simulink model "SYSTEM"  (R2026a)
settings: Solver=VariableStepAuto
model workspace (MAT data in the model file):
  CompAir_P = Simulink.ConnectionBus
  CompAir_S = Simulink.Bus
  CompAir_S.Alignment = -1
  CompAir_S.PreserveElementDimensions = 0
  CompAir_S.DataScope = 'Auto'
  Control_P = Simulink.ConnectionBus
  Control_S = Simulink.Bus
  Control_S.Alignment = -1
  Control_S.PreserveElementDimensions = 0
  Control_S.DataScope = 'Auto'
  CoolingFW_P = Simulink.ConnectionBus
  CoolingFW_S = Simulink.Bus
  CoolingFW_S.Alignment = -1
  CoolingFW_S.PreserveElementDimensions = 0
  CoolingFW_S.DataScope = 'Auto'
  FuelOil_P = Simulink.ConnectionBus
  FuelOil_S = Simulink.Bus
  FuelOil_S.Alignment = -1
  FuelOil_S.PreserveElementDimensions = 0
  FuelOil_S.DataScope = 'Auto'
  Heat_P = Simulink.ConnectionBus
  Heat_S = Simulink.Bus
  Heat_S.Alignment = -1
  Heat_S.PreserveElementDimensions = 0
  Heat_S.DataScope = 'Auto'
  LubeOil_P = Simulink.ConnectionBus
  LubeOil_S = Simulink.Bus
  LubeOil_S.Alignment = -1
  LubeOil_S.PreserveElementDimensions = 0
  LubeOil_S.DataScope = 'Auto'
  Physical = Simulink.ConnectionBus
  Power_P = Simulink.ConnectionBus
  Power_S = Simulink.Bus
  Power_S.Alignment = -1
  Power_S.PreserveElementDimensions = 0
  Power_S.DataScope = 'Auto'
  SaltWater_P = Simulink.ConnectionBus
  SaltWater_S = Simulink.Bus
  SaltWater_S.Alignment = -1
  SaltWater_S.PreserveElementDimensions = 0
  SaltWater_S.DataScope = 'Auto'
  WasteGas_P = Simulink.ConnectionBus
  WasteGas_S = Simulink.Bus
  WasteGas_S.Alignment = -1
  WasteGas_S.PreserveElementDimensions = 0
  WasteGas_S.DataScope = 'Auto'
  WasteOil_P = Simulink.ConnectionBus
  WasteOil_S = Simulink.Bus
  WasteOil_S.Alignment = -1
  WasteOil_S.PreserveElementDimensions = 0
  WasteOil_S.DataScope = 'Auto'
  WasteSolid_P = Simulink.ConnectionBus
  WasteSolid_S = Simulink.Bus
  WasteSolid_S.Alignment = -1
  WasteSolid_S.PreserveElementDimensions = 0
  WasteSolid_S.DataScope = 'Auto'
  WasteWater_P = Simulink.ConnectionBus
  WasteWater_S = Simulink.Bus
  WasteWater_S.Alignment = -1
  WasteWater_S.PreserveElementDimensions = 0
  WasteWater_S.DataScope = 'Auto'
undefined symbols (not defined in the file): FUEL
(part 1 of 5)
settings Model: VariantConfigurationObject=ConfigA  Creator=GShelton28  LastModifiedBy=sboyd

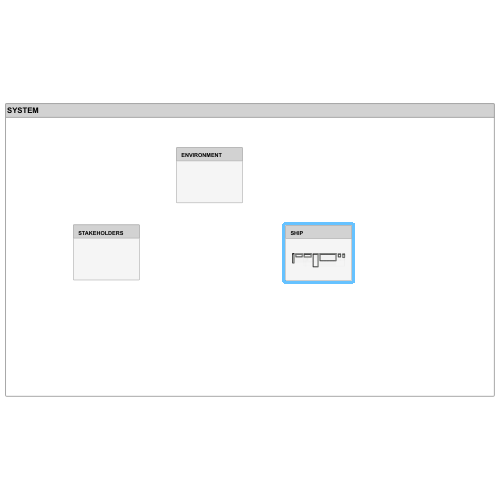
[thumbnail: Simulink's stored preview of the top-level diagram]
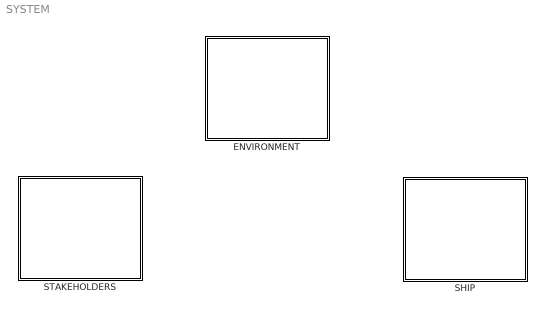
== system SYSTEM ==
  ENVIRONMENT : Subsystem
      settings: PortSchema="{\"entries\":[{\"content\":{\"headerSize\":26,\"margin\":15,\"minimumSpacing\":25,\"sides\":[{\"content\":{},\"type\":\"ConnectorPlacement.EquallySpacedRectSide\",\"uuid\":\"c62bca68-e99b-4d4a-8c3b-c9a3c6520291\"},{\"content\":{\"side\":\"RIGHT\"},\"type\":\"ConnectorPlacement.EquallySpacedRectSide\",\"uuid\":\"9f78cd75-5645-4950-8d66-9f0d33627f1f\"},{\"content\":{\"side\":\"TOP\"},\"type\":\"ConnectorPlacement.EquallySpacedRectSide\",\"uuid\":\"f95077c9-4a6b-4bf1-8b13-59697d659817\"}]},\"type\":\"ConnectorPlacement.EquallySpacedConnector\",\"uuid\":\"da1ef182-4ed3-4fb4-823f-e8eb0a5ecd15\"}],\"packageUris\":[\"http://schema.mathworks.com/mf0/Connector/R2020b\"],\"version\":\"1.0\"}"
  SHIP : Subsystem
      settings: PortSchema="{\"entries\":[{\"content\":{\"headerSize\":26,\"margin\":15,\"minimumSpacing\":25,\"sides\":[{\"content\":{},\"type\":\"ConnectorPlacement.EquallySpacedRectSide\",\"uuid\":\"c62bca68-e99b-4d4a-8c3b-c9a3c6520291\"},{\"content\":{\"side\":\"RIGHT\"},\"type\":\"ConnectorPlacement.EquallySpacedRectSide\",\"uuid\":\"9f78cd75-5645-4950-8d66-9f0d33627f1f\"},{\"content\":{\"side\":\"TOP\"},\"type\":\"ConnectorPlacement.EquallySpacedRectSide\",\"uuid\":\"f95077c9-4a6b-4bf1-8b13-59697d659817\"}]},\"type\":\"ConnectorPlacement.EquallySpacedConnector\",\"uuid\":\"da1ef182-4ed3-4fb4-823f-e8eb0a5ecd15\"}],\"packageUris\":[\"http://schema.mathworks.com/mf0/Connector/R2020b\"],\"version\":\"1.0\"}"
  STAKEHOLDERS : Subsystem
      settings: PortSchema="{\"entries\":[{\"content\":{\"headerSize\":26,\"margin\":15,\"minimumSpacing\":25,\"sides\":[{\"content\":{},\"type\":\"ConnectorPlacement.EquallySpacedRectSide\",\"uuid\":\"c62bca68-e99b-4d4a-8c3b-c9a3c6520291\"},{\"content\":{\"side\":\"RIGHT\"},\"type\":\"ConnectorPlacement.EquallySpacedRectSide\",\"uuid\":\"9f78cd75-5645-4950-8d66-9f0d33627f1f\"},{\"content\":{\"side\":\"TOP\"},\"type\":\"ConnectorPlacement.EquallySpacedRectSide\",\"uuid\":\"f95077c9-4a6b-4bf1-8b13-59697d659817\"}]},\"type\":\"ConnectorPlacement.EquallySpacedConnector\",\"uuid\":\"da1ef182-4ed3-4fb4-823f-e8eb0a5ecd15\"}],\"packageUris\":[\"http://schema.mathworks.com/mf0/Connector/R2020b\"],\"version\":\"1.0\"}"

== system SYSTEM/ENVIRONMENT ==

== system SYSTEM/SHIP ==
  100 (HULL) : Subsystem
      settings: PortSchema="{\"entries\":[{\"content\":{\"headerSize\":26,\"margin\":15,\"minimumSpacing\":25,\"sides\":[{\"content\":{},\"type\":\"ConnectorPlacement.EquallySpacedRectSide\",\"uuid\":\"c62bca68-e99b-4d4a-8c3b-c9a3c6520291\"},{\"content\":{\"connectorIds\":[\"RConn1\",\"RConn2\",\"RConn3\",\"RConn4\",\"RConn5\",\"RConn6\",\"RConn7\",\"RConn8\",\"RConn9\",\"RConn10\",\"RConn11\",\"RConn12\",\"RConn13\",\"RConn14\",\"RConn15\",\"RConn16\",\"RConn17\",\"RConn18\",\"RConn19\",\"RConn20\",\"RConn21\",\"RConn22\",\"RConn23\",\"RConn24\",\"RConn25\",\"RConn26\",\"RConn27\",\"RConn28\",\"RConn29\",\"RConn30\",\"RConn31\",\"RConn32\"],\"side\":\"RIGHT\"},\"type\":\"ConnectorPlacement.EquallySpacedRectSide\",\"uuid\":\"9f78cd75-5645-4950-8d66-9f0d33627f1f\"},{\"content\":{\"side\":\"TOP\"},\"type\":\"ConnectorPlacement.EquallySpacedRectSide\",\"uuid\":\"f95077c9-4a6b-4bf1-8b13-59697d659817\"}]},\"type\":\"ConnectorPlacement.EquallySpacedConnector\",\"uuid\":\"da1ef182-4ed3-4fb4-823f-e8eb0a5ecd15\"}],\"packageUris\":[\"http://schema.mathworks.com/mf0/Connector/R2020b\"],\"version\":\"1.0\"}"
  200 (PROPULSION) : Subsystem
      settings: PortSchema="{\"entries\":[{\"content\":{\"headerSize\":26,\"margin\":15,\"minimumSpacing\":25,\"sides\":[{\"content\":{\"connectorIds\":[\"LConn3\",\"LConn4\",\"LConn5\",\"LConn6\"]},\"type\":\"ConnectorPlacement.EquallySpacedRectSide\",\"uuid\":\"c62bca68-e99b-4d4a-8c3b-c9a3c6520291\"},{\"content\":{\"connectorIds\":[\"In11\",\"In12\",\"In13\",\"Out12\",\"Out13\",\"Out14\",\"Out15\"],\"side\":\"RIGHT\"},\"type\":\"ConnectorPlacement.EquallySpacedRectSide\",\"uuid\":\"9f78cd75-5645-4950-8d66-9f0d33627f1f\"},{\"content\":{\"connectorIds\":[\"Out1\",\"Out2\",\"Out3\",\"LConn1\",\"Out4\",\"Out5\",\"Out6\",\"Out7\",\"Out8\",\"Out9\",\"Out10\",\"Out11\",\"In1\",\"In2\",\"In3\",\"In4\",\"In5\",\"In6\",\"In7\",\"LConn2\",\"In8\",\"In9\",\"In10\"],\"side\":\"TOP\"},\"type\":\"ConnectorPlacement.EquallySpacedRectSide\",\"uuid\":\"f95077c9-4a6b-4bf1-8b13-59697d659817\"},{\"content\":{\"connectorIds\":[\"Out16\"],\"side\":\"BOTTOM\"},\"type\":\"ConnectorPlacement.EquallySpacedRectSide\",\"uuid\":\"7ad02fd3-1470-4b5e-9c8f-1c514025d559\"}]},\"type\":\"ConnectorPlacement.EquallySpacedConnector\",\"uuid\":\"da1ef182-4ed3-4fb4-823f-e8eb0a5ecd15\"}],\"packageUris\":[\"http://schema.mathworks.com/mf0/Connector/R2020b\"],\"version\":\"1.0\"}"
  300 (ELECTRICAL) : Subsystem
      settings: PortSchema="{\"entries\":[{\"content\":{\"headerSize\":26,\"margin\":15,\"minimumSpacing\":25,\"sides\":[{\"content\":{\"connectorIds\":[\"LConn3\",\"LConn4\",\"LConn5\",\"LConn6\"]},\"type\":\"ConnectorPlacement.EquallySpacedRectSide\",\"uuid\":\"c62bca68-e99b-4d4a-8c3b-c9a3c6520291\"},{\"content\":{\"connectorIds\":[\"In5\",\"In6\",\"In7\",\"In8\",\"Out6\",\"Out7\",\"Out8\",\"Out9\"],\"side\":\"RIGHT\"},\"type\":\"ConnectorPlacement.EquallySpacedRectSide\",\"uuid\":\"9f78cd75-5645-4950-8d66-9f0d33627f1f\"},{\"content\":{\"connectorIds\":[\"Out1\",\"Out2\",\"Out3\",\"LConn1\",\"Out4\",\"Out5\",\"In1\",\"In2\",\"In3\",\"LConn2\",\"In4\"],\"side\":\"TOP\"},\"type\":\"ConnectorPlacement.EquallySpacedRectSide\",\"uuid\":\"f95077c9-4a6b-4bf1-8b13-59697d659817\"},{\"content\":{\"connectorIds\":[\"In9\",\"Out10\",\"Out11\",\"Out12\",\"Out13\",\"Out14\",\"Out15\",\"Out16\",\"Out17\",\"Out18\",\"Out19\",\"Out20\",\"Out21\",\"Out22\",\"Out23\",\"Out24\",\"Out25\",\"Out26\",\"Out27\",\"Out28\",\"Out29\",\"Out30\",\"Out31\",\"Out32\"],\"side\":\"BOTTOM\"},\"type\":\"ConnectorPlacement.EquallySpacedRectSide\",\"uuid\":\"f64e9209-9b7e-40f6-99bd-cc5d8e42f30b\"}]},\"type\":\"ConnectorPlacement.EquallySpacedConnector\",\"uuid\":\"da1ef182-4ed3-4fb4-823f-e8eb0a5ecd15\"}],\"packageUris\":[\"http://schema.mathworks.com/mf0/Connector/R2020b\"],\"version\":\"1.0\"}"
  400 (COMMAND CONTROL) : Subsystem
      settings: PortSchema="{\"entries\":[{\"content\":{\"headerSize\":26,\"margin\":15,\"minimumSpacing\":25,\"sides\":[{\"content\":{\"connectorIds\":[\"LConn1\",\"LConn2\",\"LConn3\",\"LConn4\",\"LConn5\",\"LConn6\"]},\"type\":\"ConnectorPlacement.EquallySpacedRectSide\",\"uuid\":\"c62bca68-e99b-4d4a-8c3b-c9a3c6520291\"},{\"content\":{\"connectorIds\":[\"In10\",\"In11\",\"In12\",\"In13\",\"In6\",\"In7\",\"In8\",\"In9\",\"In14\",\"In15\",\"In16\",\"In17\",\"In18\",\"In19\",\"In20\",\"In21\",\"In22\",\"In23\",\"In24\",\"In25\",\"In26\",\"In27\",\"In28\",\"Out6\",\"Out7\",\"Out8\",\"Out9\",\"Out10\",\"Out11\",\"Out12\",\"Out13\",\"Out14\",\"Out15\",\"Out16\",\"Out17\",\"Out18\",\"Out19\",\"Out20\",\"Out21\",\"Out22\",\"Out23\",\"Out24\",\"Out25\",\"Out26\",\"Out27\"],\"side\":\"RIGHT\"},\"type\":\"ConnectorPlacement.EquallySpacedRectSide\",\"uuid\":\"9f78cd75-5645-4950-8d66-9f0d33627f1f\"},{\"content\":{\"connectorIds\":[\"Out1\",\"Out3\",\"Out2\",\"Out4\",\"Out5\",\"In1\",\"In3\",\"In2\",\"In4\",\"In5\"],\"side\":\"TOP\"},\"type\":\"ConnectorPlacement.EquallySpacedRectSide\",\"uuid\":\"f95077c9-4a6b-4bf1-8b13-59697d659817\"},{\"content\":{\"connectorIds\":[\"In29\",\"In30\",\"In31\",\"In32\",\"In33\",\"In34\"],\"side\":\"BOTTOM\"},\"type\":\"ConnectorPlacement.EquallySpacedRectSide\",\"uuid\":\"b87ed66e-141b-41a3-a484-184f926198b1\"}]},\"type\":\"ConnectorPlacement.EquallySpacedConnector\",\"uuid\":\"da1ef182-4ed3-4fb4-823f-e8eb0a5ecd15\"}],\"packageUris\":[\"http://schema.mathworks.com/mf0/Connector/R2020b\"],\"version\":\"1.0\"}"
  500 (AUXILLIARY SYSTEMS) : Subsystem
      settings: PortSchema="{\"entries\":[{\"content\":{\"headerSize\":26,\"margin\":15,\"minimumSpacing\":25,\"sides\":[{\"content\":{\"connectorIds\":[\"LConn5\",\"LConn6\",\"LConn7\",\"LConn8\",\"LConn9\",\"LConn10\",\"LConn11\",\"LConn12\",\"LConn13\",\"LConn14\"]},\"type\":\"ConnectorPlacement.EquallySpacedRectSide\",\"uuid\":\"c62bca68-e99b-4d4a-8c3b-c9a3c6520291\"},{\"content\":{\"connectorIds\":[\"In31\",\"In32\",\"In33\",\"In34\",\"In35\",\"In36\",\"In37\",\"In38\",\"In39\",\"In40\",\"In41\",\"In42\",\"Out25\",\"Out26\",\"Out27\",\"Out28\",\"Out29\",\"Out30\",\"Out31\",\"Out32\",\"Out33\",\"Out34\",\"Out35\",\"Out36\"],\"side\":\"RIGHT\"},\"type\":\"ConnectorPlacement.EquallySpacedRectSide\",\"uuid\":\"9f78cd75-5645-4950-8d66-9f0d33627f1f\"},{\"content\":{\"connectorIds\":[\"Out1\",\"Out2\",\"Out3\",\"Out4\",\"Out5\",\"Out6\",\"Out7\",\"Out8\",\"Out9\",\"Out10\",\"Out11\",\"Out12\",\"Out13\",\"Out14\",\"Out15\",\"Out16\",\"Out17\",\"Out18\",\"LConn1\",\"Out19\",\"LConn2\",\"Out20\",\"Out21\",\"Out22\",\"Out23\",\"Out24\",\"In1\",\"In25\",\"In3\",\"LConn3\",\"In4\",\"In5\",\"In2\",\"In28\",\"In8\",\"In29\",\"In10\",\"In30\",\"In6\",\"In13\",\"In14\",\"LConn4\",\"In15\",\"In16\",\"In17\",\"In7\",\"In9\",\"In20\",\"In11\",\"In12\",\"In23\",\"In24\",\"In22\",\"In26\",\"In27\",\"In19\",\"In21\",\"In18\"],\"side\":\"TOP\"},\"type\":\"ConnectorPlacement.EquallySpacedRectSide\",\"uuid\":\"f95077c9-4a6b-4bf1-8b13-59697d659817\"},{\"content\":{\"connectorIds\":[\"In43\",\"In44\",\"In45\",\"In46\",\"In47\",\"In48\",\"In49\",\"In50\",\"In51\",\"In52\"],\"side\":\"BOTTOM\"},\"type\":\"ConnectorPlacement.EquallySpacedRectSide\",\"uuid\":\"1e4b81d9-ad89-4d5a-adb7-9dee60647f33\"}]},\"type\":\"ConnectorPlacement.EquallySpacedConnector\",\"uuid\":\"da1ef182-4ed3-4fb4-823f-e8eb0a5ecd15\"}],\"packageUris\":[\"http://schema.mathworks.com/mf0/Connector/R2020b\"],\"version\":\"1.0\"}"
  600 (OUTFITTING) : Subsystem
      settings: PortSchema="{\"entries\":[{\"content\":{\"headerSize\":26,\"margin\":15,\"minimumSpacing\":25,\"sides\":[{\"content\":{\"connectorIds\":[\"LConn1\",\"LConn2\",\"LConn3\"]},\"type\":\"ConnectorPlacement.EquallySpacedRectSide\",\"uuid\":\"c62bca68-e99b-4d4a-8c3b-c9a3c6520291\"},{\"content\":{\"connectorIds\":[\"In3\",\"In4\",\"Out7\",\"Out8\"],\"side\":\"RIGHT\"},\"type\":\"ConnectorPlacement.EquallySpacedRectSide\",\"uuid\":\"9f78cd75-5645-4950-8d66-9f0d33627f1f\"},{\"content\":{\"connectorIds\":[\"Out1\",\"Out2\",\"Out3\",\"Out4\",\"Out5\",\"Out6\",\"In1\",\"In2\"],\"side\":\"TOP\"},\"type\":\"ConnectorPlacement.EquallySpacedRectSide\",\"uuid\":\"f95077c9-4a6b-4bf1-8b13-59697d659817\"},{\"content\":{\"connectorIds\":[\"In5\",\"In6\"],\"side\":\"BOTTOM\"},\"type\":\"ConnectorPlacement.EquallySpacedRectSide\",\"uuid\":\"1c2b3604-2b1a-4429-bb6b-614e1a01ce36\"}]},\"type\":\"ConnectorPlacement.EquallySpacedConnector\",\"uuid\":\"da1ef182-4ed3-4fb4-823f-e8eb0a5ecd15\"}],\"packageUris\":[\"http://schema.mathworks.com/mf0/Connector/R2020b\"],\"version\":\"1.0\"}"
  700 (WEAPONS) : Subsystem
      settings: PortSchema="{\"entries\":[{\"content\":{\"headerSize\":26,\"margin\":15,\"minimumSpacing\":25,\"sides\":[{\"content\":{\"connectorIds\":[\"LConn1\",\"LConn2\",\"LConn3\",\"LConn4\",\"LConn5\"]},\"type\":\"ConnectorPlacement.EquallySpacedRectSide\",\"uuid\":\"c62bca68-e99b-4d4a-8c3b-c9a3c6520291\"},{\"content\":{\"connectorIds\":[\"In4\",\"In5\",\"In6\",\"In7\",\"In8\",\"Out4\",\"Out5\",\"Out6\",\"Out7\",\"Out8\"],\"side\":\"RIGHT\"},\"type\":\"ConnectorPlacement.EquallySpacedRectSide\",\"uuid\":\"9f78cd75-5645-4950-8d66-9f0d33627f1f\"},{\"content\":{\"connectorIds\":[\"Out1\",\"Out2\",\"Out3\",\"In1\",\"In2\",\"In3\"],\"side\":\"TOP\"},\"type\":\"ConnectorPlacement.EquallySpacedRectSide\",\"uuid\":\"f95077c9-4a6b-4bf1-8b13-59697d659817\"},{\"content\":{\"connectorIds\":[\"In9\",\"In10\",\"In11\",\"In12\",\"In13\"],\"side\":\"BOTTOM\"},\"type\":\"ConnectorPlacement.EquallySpacedRectSide\",\"uuid\":\"b18ac05c-61d0-41e7-b1c6-0cdd3a4fef39\"}]},\"type\":\"ConnectorPlacement.EquallySpacedConnector\",\"uuid\":\"da1ef182-4ed3-4fb4-823f-e8eb0a5ecd15\"}],\"packageUris\":[\"http://schema.mathworks.com/mf0/Connector/R2020b\"],\"version\":\"1.0\"}"
  wires:
  200 (PROPULSION)/16(23X-31XP) -> 300 (ELECTRICAL)/9(23X-31XP)
  300 (ELECTRICAL)/10(31X-40XP) -> 400 (COMMAND CONTROL)/29(31X-40XP)
  300 (ELECTRICAL)/11(31X-41XP) -> 400 (COMMAND CONTROL)/30(31X-41XP)
  300 (ELECTRICAL)/12(31X-42XP) -> 400 (COMMAND CONTROL)/31(31X-42XP)
  300 (ELECTRICAL)/13(31X-43XP) -> 400 (COMMAND CONTROL)/32(31X-43XP)
  300 (ELECTRICAL)/14(31X-44XP) -> 400 (COMMAND CONTROL)/33(31X-44XP)
  300 (ELECTRICAL)/15(31X-45XP) -> 400 (COMMAND CONTROL)/34(31X-45XP)
  300 (ELECTRICAL)/16(31X-50XP) -> 500 (AUXILLIARY SYSTEMS)/43(31X-50XP)
  300 (ELECTRICAL)/17(31X-51XP) -> 500 (AUXILLIARY SYSTEMS)/44(31X-51XP)
  300 (ELECTRICAL)/18(31X-529P) -> 500 (AUXILLIARY SYSTEMS)/45(31X-529P)
  300 (ELECTRICAL)/19(31X-53XP) -> 500 (AUXILLIARY SYSTEMS)/46(31X-53XP)
  300 (ELECTRICAL)/20(31X-54XP) -> 500 (AUXILLIARY SYSTEMS)/47(31X-54XP)
  300 (ELECTRICAL)/21(31X-55XP) -> 500 (AUXILLIARY SYSTEMS)/48(31X-55XP)
  300 (ELECTRICAL)/22(31X-56XP) -> 500 (AUXILLIARY SYSTEMS)/49(31X-56XP)
  300 (ELECTRICAL)/23(31X-57XP) -> 500 (AUXILLIARY SYSTEMS)/50(31X-57XP)
  300 (ELECTRICAL)/24(31X-58XP) -> 500 (AUXILLIARY SYSTEMS)/51(31X-58XP)
  300 (ELECTRICAL)/25(31X-59XP) -> 500 (AUXILLIARY SYSTEMS)/52(31X-59XP)
  300 (ELECTRICAL)/26(31X-60XP) -> 600 (OUTFITTING)/5(31X-60XP)
  300 (ELECTRICAL)/27(31X-61XP) -> 600 (OUTFITTING)/6(31X-61XP)
  300 (ELECTRICAL)/28(31X-70XP) -> 700 (WEAPONS)/9(31X-70XP)
  300 (ELECTRICAL)/29(31X-71XP) -> 700 (WEAPONS)/10(31X-71XP)
  300 (ELECTRICAL)/30(31X-72XP) -> 700 (WEAPONS)/11(31X-72XP)
  300 (ELECTRICAL)/31(31X-73XP) -> 700 (WEAPONS)/12(31X-73XP)
  300 (ELECTRICAL)/32(31X-74XP) -> 700 (WEAPONS)/13(31X-74XP)
  200 (PROPULSION)/12(20X-42XC) -> 400 (COMMAND CONTROL)/10(20X-42XC)
  200 (PROPULSION)/13(21X-42XC) -> 400 (COMMAND CONTROL)/11(21X-42XC)
  200 (PROPULSION)/15(23X-42XC) -> 400 (COMMAND CONTROL)/13(23X-42XC)
  400 (COMMAND CONTROL)/6(42X-20XC) -> 200 (PROPULSION)/11(42X-20XC)
  400 (COMMAND CONTROL)/7(42X-21XC) -> 200 (PROPULSION)/12(42X-21XC)
  400 (COMMAND CONTROL)/8(42X-23XC) -> 200 (PROPULSION)/13(42X-23XC)
  200 (PROPULSION)/14(22X-42XC) -> 400 (COMMAND CONTROL)/12(22X-42XC)
  400 (COMMAND CONTROL)/9(42X-30XC) -> 300 (ELECTRICAL)/5(42X-30XC)
  400 (COMMAND CONTROL)/10(42X-31XC) -> 300 (ELECTRICAL)/6(42X-31XC)
  400 (COMMAND CONTROL)/11(42X-32XC) -> 300 (ELECTRICAL)/7(42X-32XC)
  400 (COMMAND CONTROL)/12(42X-33XC) -> 300 (ELECTRICAL)/8(42X-33XC)
  300 (ELECTRICAL)/6(30X-42XC) -> 400 (COMMAND CONTROL)/6(30X-42XC)
  300 (ELECTRICAL)/7(31X-42XC) -> 400 (COMMAND CONTROL)/7(31X-42XC)
  300 (ELECTRICAL)/8(32X-42XC) -> 400 (COMMAND CONTROL)/8(32X-42XC)
  300 (ELECTRICAL)/9(33X-42XC) -> 400 (COMMAND CONTROL)/9(33X-42XC)
  500 (AUXILLIARY SYSTEMS)/25(50X-42XC) -> 400 (COMMAND CONTROL)/14(50X-42XC)
  500 (AUXILLIARY SYSTEMS)/26(51X-42XC) -> 400 (COMMAND CONTROL)/15(51X-42XC)
  500 (AUXILLIARY SYSTEMS)/27(528-42XC) -> 400 (COMMAND CONTROL)/16(528-42XC)
  500 (AUXILLIARY SYSTEMS)/28(53X-42XC) -> 400 (COMMAND CONTROL)/17(53X-42XC)
  500 (AUXILLIARY SYSTEMS)/29(54X-42XC) -> 400 (COMMAND CONTROL)/18(54X-42XC)
  500 (AUXILLIARY SYSTEMS)/30(55X-42XC) -> 400 (COMMAND CONTROL)/19(55X-42XC)
  500 (AUXILLIARY SYSTEMS)/31(56X-42XC) -> 400 (COMMAND CONTROL)/20(56X-42XC)
  500 (AUXILLIARY SYSTEMS)/32(57X-42XC) -> 400 (COMMAND CONTROL)/21(57X-42XC)
  500 (AUXILLIARY SYSTEMS)/33(58X-42XC) -> 400 (COMMAND CONTROL)/22(58X-42XC)
  500 (AUXILLIARY SYSTEMS)/34(59X-42XC) -> 400 (COMMAND CONTROL)/23(59X-42XC)
  400 (COMMAND CONTROL)/13(42X-50XC) -> 500 (AUXILLIARY SYSTEMS)/31(42X-50XC)
  400 (COMMAND CONTROL)/14(42X-51XC) -> 500 (AUXILLIARY SYSTEMS)/32(42X-51XC)
  400 (COMMAND CONTROL)/15(42X-528C) -> 500 (AUXILLIARY SYSTEMS)/33(42X-528C)
  400 (COMMAND CONTROL)/16(42X-53XC) -> 500 (AUXILLIARY SYSTEMS)/34(42X-53XC)
  400 (COMMAND CONTROL)/17(42X-54XC) -> 500 (AUXILLIARY SYSTEMS)/35(42X-54XC)
  400 (COMMAND CONTROL)/18(42X-55XC) -> 500 (AUXILLIARY SYSTEMS)/36(42X-55XC)
  400 (COMMAND CONTROL)/19(42X-56XC) -> 500 (AUXILLIARY SYSTEMS)/37(42X-56XC)
  400 (COMMAND CONTROL)/20(42X-57XC) -> 500 (AUXILLIARY SYSTEMS)/38(42X-57XC)
  400 (COMMAND CONTROL)/21(42X-58XC) -> 500 (AUXILLIARY SYSTEMS)/39(42X-58XC)
  400 (COMMAND CONTROL)/22(42X-59XC) -> 500 (AUXILLIARY SYSTEMS)/40(42X-59XC)
  700 (WEAPONS)/4(70X-42XC) -> 400 (COMMAND CONTROL)/24(70X-42XC)
  700 (WEAPONS)/5(71X-42XC) -> 400 (COMMAND CONTROL)/25(71X-42XC)
  700 (WEAPONS)/6(72X-42XC) -> 400 (COMMAND CONTROL)/26(72X-42XC)
  700 (WEAPONS)/7(73X-42XC) -> 400 (COMMAND CONTROL)/27(73X-42XC)
  700 (WEAPONS)/8(74X-42XC) -> 400 (COMMAND CONTROL)/28(74X-42XC)
  400 (COMMAND CONTROL)/23(42X-70XC) -> 700 (WEAPONS)/4(42X-70XC)
  400 (COMMAND CONTROL)/24(42X-71XC) -> 700 (WEAPONS)/5(42X-71XC)
  400 (COMMAND CONTROL)/25(42X-72XC) -> 700 (WEAPONS)/6(42X-72XC)
  400 (COMMAND CONTROL)/26(42X-73XC) -> 700 (WEAPONS)/7(42X-73XC)
  400 (COMMAND CONTROL)/27(42X-74XC) -> 700 (WEAPONS)/8(42X-74XC)
  600 (OUTFITTING)/7(60X-59XC) -> 500 (AUXILLIARY SYSTEMS)/41(60X-59XC)
  600 (OUTFITTING)/8(61X-59XC) -> 500 (AUXILLIARY SYSTEMS)/42(61X-59XC)
  500 (AUXILLIARY SYSTEMS)/35(59X-60XC) -> 600 (OUTFITTING)/3(59X-60XC)
  500 (AUXILLIARY SYSTEMS)/36(59X-61XC) -> 600 (OUTFITTING)/4(59X-61XC)
  500 (AUXILLIARY SYSTEMS)/1(50X-20XCFW) -> 200 (PROPULSION)/1(50X-20XCFW)
  500 (AUXILLIARY SYSTEMS)/2(50X-21XCFW) -> 200 (PROPULSION)/2(50X-21XCFW)
  200 (PROPULSION)/1(20X-50XCFW) -> 500 (AUXILLIARY SYSTEMS)/1(20X-50XCFW)
  200 (PROPULSION)/6(21X-50XCFW) -> 500 (AUXILLIARY SYSTEMS)/2(21X-50XCFW)
  300 (ELECTRICAL)/1(30X-50XCFW) -> 500 (AUXILLIARY SYSTEMS)/6(30X-50XCFW)
  500 (AUXILLIARY SYSTEMS)/3(50X-30XCFW) -> 300 (ELECTRICAL)/1(50X-30XCFW)
  400 (COMMAND CONTROL)/2(43X-50XCFW) -> 500 (AUXILLIARY SYSTEMS)/9(43X-50XCFW)
  500 (AUXILLIARY SYSTEMS)/5(50X-43XCFW) -> 400 (COMMAND CONTROL)/3(50X-43XCFW)
  500 (AUXILLIARY SYSTEMS)/4(50X-42XCFW) -> 400 (COMMAND CONTROL)/1(50X-42XCFW)
  500 (AUXILLIARY SYSTEMS)/6(50X-44XCFW) -> 400 (COMMAND CONTROL)/2(50X-44XCFW)
  400 (COMMAND CONTROL)/5(44X-50XCFW) -> 500 (AUXILLIARY SYSTEMS)/11(44X-50XCFW)
  400 (COMMAND CONTROL)/3(42X-50XCFW) -> 500 (AUXILLIARY SYSTEMS)/7(42X-50XCFW)
  600 (OUTFITTING)/1(60X-50XCFW) -> 500 (AUXILLIARY SYSTEMS)/12(60X-50XCFW)
  600 (OUTFITTING)/4(61X-50XCFW) -> 500 (AUXILLIARY SYSTEMS)/22(61X-50XCFW)
  500 (AUXILLIARY SYSTEMS)/7(50X-60XCFW) -> 600 (OUTFITTING)/1(50X-60XCFW)
  500 (AUXILLIARY SYSTEMS)/8(50X-61XCFW) -> 600 (OUTFITTING)/2(50X-61XCFW)
  700 (WEAPONS)/3(73X-50XCFW) -> 500 (AUXILLIARY SYSTEMS)/18(73X-50XCFW)
  700 (WEAPONS)/2(72X-50XCFW) -> 500 (AUXILLIARY SYSTEMS)/21(72X-50XCFW)
  700 (WEAPONS)/1(71X-50XCFW) -> 500 (AUXILLIARY SYSTEMS)/19(71X-50XCFW)
  500 (AUXILLIARY SYSTEMS)/9(50X-71XCFW) -> 700 (WEAPONS)/1(50X-71XCFW)
  500 (AUXILLIARY SYSTEMS)/10(50X-72XCFW) -> 700 (WEAPONS)/2(50X-72XCFW)
  500 (AUXILLIARY SYSTEMS)/11(50X-73XCFW) -> 700 (WEAPONS)/3(50X-73XCFW)
  500 (AUXILLIARY SYSTEMS)/12(51X-20XLO) -> 200 (PROPULSION)/3(51X-20XLO)
  500 (AUXILLIARY SYSTEMS)/13(51X-21XLO) -> 200 (PROPULSION)/4(51X-21XLO)
  500 (AUXILLIARY SYSTEMS)/14(51X-22XLO) -> 200 (PROPULSION)/5(51X-22XLO)
  500 (AUXILLIARY SYSTEMS)/15(51X-23XLO) -> 200 (PROPULSION)/6(51X-23XLO)
  200 (PROPULSION)/2(20X-51XLO) -> 500 (AUXILLIARY SYSTEMS)/25(20X-51XLO)
  200 (PROPULSION)/7(21X-51XLO) -> 500 (AUXILLIARY SYSTEMS)/28(21X-51XLO)
  200 (PROPULSION)/9(22X-51XLO) -> 500 (AUXILLIARY SYSTEMS)/29(22X-51XLO)
  200 (PROPULSION)/11(23X-51XLO) -> 500 (AUXILLIARY SYSTEMS)/30(23X-51XLO)
  300 (ELECTRICAL)/2(30X-51XLO) -> 500 (AUXILLIARY SYSTEMS)/13(30X-51XLO)
  500 (AUXILLIARY SYSTEMS)/16(51X-30XLO) -> 300 (ELECTRICAL)/2(51X-30XLO)
  500 (AUXILLIARY SYSTEMS)/17(51X-43XLO) -> 400 (COMMAND CONTROL)/4(51X-43XLO)
  400 (COMMAND CONTROL)/4(43X-51XLO) -> 500 (AUXILLIARY SYSTEMS)/20(43X-51XLO)
  200 (PROPULSION)/3(20X-52XFO) -> 500 (AUXILLIARY SYSTEMS)/3(20X-52XFO)
  500 (AUXILLIARY SYSTEMS)/18(52X-20XFO) -> 200 (PROPULSION)/7(52X-20XFO)
  300 (ELECTRICAL)/3(30X-52XFO) -> 500 (AUXILLIARY SYSTEMS)/14(30X-52XFO)
  500 (AUXILLIARY SYSTEMS)/19(52X-30XFO) -> 300 (ELECTRICAL)/3(52X-30XFO)
  500 (AUXILLIARY SYSTEMS)/20(53X-20XCA) -> 200 (PROPULSION)/8(53X-20XCA)
  500 (AUXILLIARY SYSTEMS)/21(53X-21XCA) -> 200 (PROPULSION)/9(53X-21XCA)
  500 (AUXILLIARY SYSTEMS)/22(53X-22XCA) -> 200 (PROPULSION)/10(53X-22XCA)
  200 (PROPULSION)/4(20X-53XCA) -> 500 (AUXILLIARY SYSTEMS)/4(20X-53XCA)
  200 (PROPULSION)/8(21X-53XCA) -> 500 (AUXILLIARY SYSTEMS)/8(21X-53XCA)
  200 (PROPULSION)/10(22X-53XCA) -> 500 (AUXILLIARY SYSTEMS)/10(22X-53XCA)
  500 (AUXILLIARY SYSTEMS)/23(53X-30XCA) -> 300 (ELECTRICAL)/4(53X-30XCA)
  300 (ELECTRICAL)/4(30X-53XCA) -> 500 (AUXILLIARY SYSTEMS)/15(30X-53XCA)
  500 (AUXILLIARY SYSTEMS)/24(53X-40XCA) -> 400 (COMMAND CONTROL)/5(53X-40XCA)
  400 (COMMAND CONTROL)/1(40X-53XCA) -> 500 (AUXILLIARY SYSTEMS)/17(40X-53XCA)
  600 (OUTFITTING)/2(60X-57XWW) -> 500 (AUXILLIARY SYSTEMS)/23(60X-57XWW)
  600 (OUTFITTING)/5(61X-57XWW) -> 500 (AUXILLIARY SYSTEMS)/26(61X-57XWW)
  600 (OUTFITTING)/3(60X-57XWS) -> 500 (AUXILLIARY SYSTEMS)/24(60X-57XWS)
  600 (OUTFITTING)/6(61X-57XWS) -> 500 (AUXILLIARY SYSTEMS)/27(61X-57XWS)
  300 (ELECTRICAL)/5(30X-57XWG) -> 500 (AUXILLIARY SYSTEMS)/16(30X-57XWG)
  200 (PROPULSION)/5(20X-57XWG) -> 500 (AUXILLIARY SYSTEMS)/5(20X-57XWG)
  connections:
  200 (PROPULSION)/LConn3 -- 100 (HULL)/RConn1
  200 (PROPULSION)/LConn4 -- 100 (HULL)/RConn2
  200 (PROPULSION)/LConn5 -- 100 (HULL)/RConn3
  200 (PROPULSION)/LConn6 -- 100 (HULL)/RConn4
  300 (ELECTRICAL)/LConn3 -- 100 (HULL)/RConn5
  300 (ELECTRICAL)/LConn4 -- 100 (HULL)/RConn6
  300 (ELECTRICAL)/LConn5 -- 100 (HULL)/RConn7
  300 (ELECTRICAL)/LConn6 -- 100 (HULL)/RConn8
  400 (COMMAND CONTROL)/LConn1 -- 100 (HULL)/RConn9
  400 (COMMAND CONTROL)/LConn2 -- 100 (HULL)/RConn10
  400 (COMMAND CONTROL)/LConn3 -- 100 (HULL)/RConn11
  400 (COMMAND CONTROL)/LConn4 -- 100 (HULL)/RConn12
  400 (COMMAND CONTROL)/LConn5 -- 100 (HULL)/RConn13
  400 (COMMAND CONTROL)/LConn6 -- 100 (HULL)/RConn14
  500 (AUXILLIARY SYSTEMS)/LConn5 -- 100 (HULL)/RConn15
  500 (AUXILLIARY SYSTEMS)/LConn6 -- 100 (HULL)/RConn16
  500 (AUXILLIARY SYSTEMS)/LConn7 -- 100 (HULL)/RConn17
  500 (AUXILLIARY SYSTEMS)/LConn8 -- 100 (HULL)/RConn18
  500 (AUXILLIARY SYSTEMS)/LConn9 -- 100 (HULL)/RConn19
  500 (AUXILLIARY SYSTEMS)/LConn10 -- 100 (HULL)/RConn20
  500 (AUXILLIARY SYSTEMS)/LConn11 -- 100 (HULL)/RConn21
  500 (AUXILLIARY SYSTEMS)/LConn12 -- 100 (HULL)/RConn22
  500 (AUXILLIARY SYSTEMS)/LConn13 -- 100 (HULL)/RConn23
  500 (AUXILLIARY SYSTEMS)/LConn14 -- 100 (HULL)/RConn24
  600 (OUTFITTING)/LConn1 -- 100 (HULL)/RConn25
  600 (OUTFITTING)/LConn2 -- 100 (HULL)/RConn26
  600 (OUTFITTING)/LConn3 -- 100 (HULL)/RConn27
  700 (WEAPONS)/LConn1 -- 100 (HULL)/RConn28
  100 (HULL)/RConn29 -- 700 (WEAPONS)/LConn2
  700 (WEAPONS)/LConn3 -- 100 (HULL)/RConn30
  100 (HULL)/RConn31 -- 700 (WEAPONS)/LConn4
  700 (WEAPONS)/LConn5 -- 100 (HULL)/RConn32
  500 (AUXILLIARY SYSTEMS)/LConn1 -- 200 (PROPULSION)/LConn2
  500 (AUXILLIARY SYSTEMS)/LConn3 -- 200 (PROPULSION)/LConn1
  500 (AUXILLIARY SYSTEMS)/LConn2 -- 300 (ELECTRICAL)/LConn2
  500 (AUXILLIARY SYSTEMS)/LConn4 -- 300 (ELECTRICAL)/LConn1

== system SYSTEM/STAKEHOLDERS ==

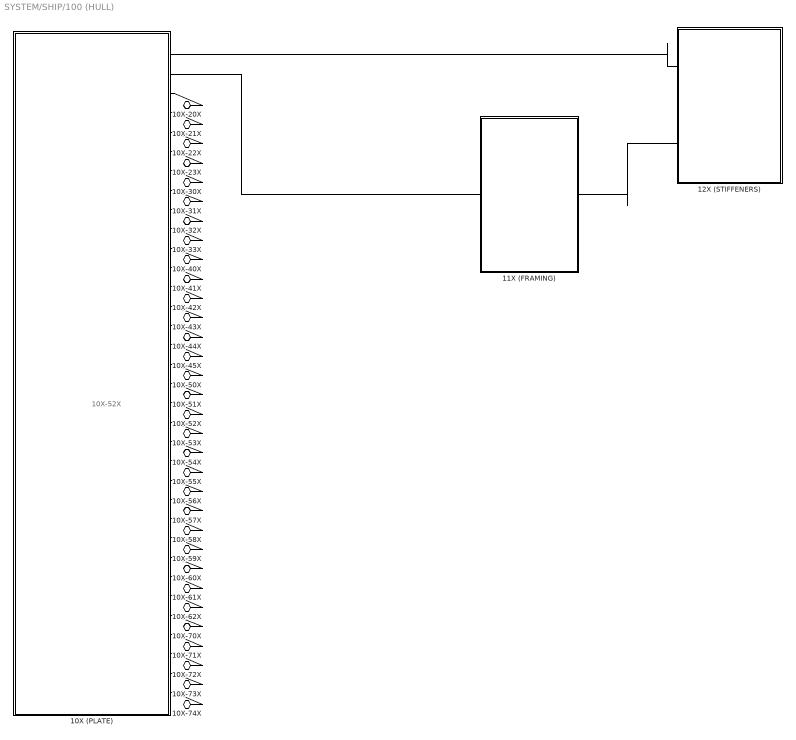
== system SYSTEM/SHIP/100 (HULL) ==
  note: 10X-52X
  10X (PLATE) : Subsystem
      settings: PortSchema="{\"entries\":[{\"content\":{\"headerSize\":26,\"margin\":15,\"minimumSpacing\":25,\"sides\":[{\"content\":{},\"type\":\"ConnectorPlacement.EquallySpacedRectSide\",\"uuid\":\"c62bca68-e99b-4d4a-8c3b-c9a3c6520291\"},{\"content\":{\"connectorIds\":[\"RConn1\",\"RConn2\",\"RConn3\",\"RConn4\",\"RConn5\",\"RConn6\",\"RConn7\",\"RConn8\",\"RConn9\",\"RConn10\",\"RConn11\",\"RConn12\",\"RConn13\",\"RConn14\",\"RConn15\",\"RConn16\",\"RConn17\",\"RConn18\",\"RConn19\",\"RConn20\",\"RConn21\",\"RConn22\",\"RConn23\",\"RConn24\",\"RConn25\",\"RConn26\",\"RConn27\",\"RConn28\",\"RConn29\",\"RConn30\",\"RConn31\",\"RConn32\",\"RConn33\",\"RConn34\"],\"side\":\"RIGHT\"},\"type\":\"ConnectorPlacement.EquallySpacedRectSide\",\"uuid\":\"9f78cd75-5645-4950-8d66-9f0d33627f1f\"},{\"content\":{\"side\":\"TOP\"},\"type\":\"ConnectorPlacement.EquallySpacedRectSide\",\"uuid\":\"f95077c9-4a6b-4bf1-8b13-59697d659817\"},{\"content\":{\"side\":\"BOTTOM\"},\"type\":\"ConnectorPlacement.EquallySpacedRectSide\",\"uuid\":\"ddd19866-59cb-4aa8-acfa-d5f465b87cbd\"}]},\"type\":\"ConnectorPlacement.EquallySpacedConnector\",\"uuid\":\"da1ef182-4ed3-4fb4-823f-e8eb0a5ecd15\"}],\"packageUris\":[\"http://schema.mathworks.com/mf0/Connector/R2020b\"],\"version\":\"1.0\"}"
  11X (FRAMING) : Subsystem
      settings: PortSchema="{\"entries\":[{\"content\":{\"headerSize\":26,\"margin\":15,\"minimumSpacing\":25,\"sides\":[{\"content\":{\"connectorIds\":[\"LConn1\"]},\"type\":\"ConnectorPlacement.EquallySpacedRectSide\",\"uuid\":\"c62bca68-e99b-4d4a-8c3b-c9a3c6520291\"},{\"content\":{\"connectorIds\":[\"RConn1\"],\"side\":\"RIGHT\"},\"type\":\"ConnectorPlacement.EquallySpacedRectSide\",\"uuid\":\"9f78cd75-5645-4950-8d66-9f0d33627f1f\"},{\"content\":{\"side\":\"TOP\"},\"type\":\"ConnectorPlacement.EquallySpacedRectSide\",\"uuid\":\"f95077c9-4a6b-4bf1-8b13-59697d659817\"},{\"content\":{\"side\":\"BOTTOM\"},\"type\":\"ConnectorPlacement.EquallySpacedRectSide\",\"uuid\":\"e30eef64-4d31-47ea-aab5-fe3e5ba0a546\"}]},\"type\":\"ConnectorPlacement.EquallySpacedConnector\",\"uuid\":\"da1ef182-4ed3-4fb4-823f-e8eb0a5ecd15\"}],\"packageUris\":[\"http://schema.mathworks.com/mf0/Connector/R2020b\"],\"version\":\"1.0\"}"
  12X (STIFFENERS) : Subsystem
      settings: PortSchema="{\"entries\":[{\"content\":{\"headerSize\":26,\"margin\":15,\"minimumSpacing\":25,\"sides\":[{\"content\":{\"connectorIds\":[\"LConn1\",\"LConn2\"]},\"type\":\"ConnectorPlacement.EquallySpacedRectSide\",\"uuid\":\"c62bca68-e99b-4d4a-8c3b-c9a3c6520291\"},{\"content\":{\"side\":\"RIGHT\"},\"type\":\"ConnectorPlacement.EquallySpacedRectSide\",\"uuid\":\"9f78cd75-5645-4950-8d66-9f0d33627f1f\"},{\"content\":{\"side\":\"TOP\"},\"type\":\"ConnectorPlacement.EquallySpacedRectSide\",\"uuid\":\"f95077c9-4a6b-4bf1-8b13-59697d659817\"},{\"content\":{\"side\":\"BOTTOM\"},\"type\":\"ConnectorPlacement.EquallySpacedRectSide\",\"uuid\":\"7faf6a59-0ecd-4c67-a0ee-65a3195c0019\"}]},\"type\":\"ConnectorPlacement.EquallySpacedConnector\",\"uuid\":\"da1ef182-4ed3-4fb4-823f-e8eb0a5ecd15\"}],\"packageUris\":[\"http://schema.mathworks.com/mf0/Connector/R2020b\"],\"version\":\"1.0\"}"
  10X-20X : PMIOPort  Side=Right  ConnectionType=Bus: Physical
  10X-21X : PMIOPort  Port=2  Side=Right  ConnectionType=Bus: Physical
  10X-22X : PMIOPort  Port=3  Side=Right  ConnectionType=Bus: Physical
  10X-23X : PMIOPort  Port=4  Side=Right  ConnectionType=Bus: Physical
  10X-30X : PMIOPort  Port=5  Side=Right  ConnectionType=Bus: Physical
  10X-31X : PMIOPort  Port=6  Side=Right  ConnectionType=Bus: Physical
  10X-32X : PMIOPort  Port=7  Side=Right  ConnectionType=Bus: Physical
  10X-33X : PMIOPort  Port=8  Side=Right  ConnectionType=Bus: Physical
  10X-40X : PMIOPort  Port=9  Side=Right  ConnectionType=Bus: Physical
  10X-41X : PMIOPort  Port=10  Side=Right  ConnectionType=Bus: Physical
  10X-42X : PMIOPort  Port=11  Side=Right  ConnectionType=Bus: Physical
  10X-43X : PMIOPort  Port=12  Side=Right  ConnectionType=Bus: Physical
  10X-44X : PMIOPort  Port=13  Side=Right  ConnectionType=Bus: Physical
  10X-45X : PMIOPort  Port=14  Side=Right  ConnectionType=Bus: Physical
  10X-50X : PMIOPort  Port=15  Side=Right  ConnectionType=Bus: Physical
  10X-51X : PMIOPort  Port=16  Side=Right  ConnectionType=Bus: Physical
  10X-52X : PMIOPort  Port=17  Side=Right  ConnectionType=Bus: Physical
  10X-53X : PMIOPort  Port=18  Side=Right  ConnectionType=Bus: Physical
  10X-54X : PMIOPort  Port=19  Side=Right  ConnectionType=Bus: Physical
  10X-55X : PMIOPort  Port=20  Side=Right  ConnectionType=Bus: Physical
  10X-56X : PMIOPort  Port=21  Side=Right  ConnectionType=Bus: Physical
  10X-57X : PMIOPort  Port=22  Side=Right  ConnectionType=Bus: Physical
  10X-58X : PMIOPort  Port=23  Side=Right  ConnectionType=Bus: Physical
  10X-59X : PMIOPort  Port=24  Side=Right  ConnectionType=Bus: Physical
  10X-60X : PMIOPort  Port=25  Side=Right  ConnectionType=Bus: Physical
  10X-61X : PMIOPort  Port=26  Side=Right  ConnectionType=Bus: Physical
  10X-62X : PMIOPort  Port=27  Side=Right  ConnectionType=Bus: Physical
  10X-70X : PMIOPort  Port=28  Side=Right  ConnectionType=Bus: Physical
  10X-71X : PMIOPort  Port=29  Side=Right  ConnectionType=Bus: Physical
  10X-72X : PMIOPort  Port=30  Side=Right  ConnectionType=Bus: Physical
  10X-73X : PMIOPort  Port=31  Side=Right  ConnectionType=Bus: Physical
  10X-74X : PMIOPort  Port=32  Side=Right  ConnectionType=Bus: Physical
  connections:
  10X (PLATE)/RConn2 -- 11X (FRAMING)/LConn1
  12X (STIFFENERS)/LConn2 -- 11X (FRAMING)/RConn1
  12X (STIFFENERS)/LConn1 -- 10X (PLATE)/RConn1
  10X-20X/RConn1 -- 10X (PLATE)/RConn3
  10X-21X/RConn1 -- 10X (PLATE)/RConn4
  10X-22X/RConn1 -- 10X (PLATE)/RConn5
  10X-23X/RConn1 -- 10X (PLATE)/RConn6
  10X-30X/RConn1 -- 10X (PLATE)/RConn7
  10X-31X/RConn1 -- 10X (PLATE)/RConn8
  10X-32X/RConn1 -- 10X (PLATE)/RConn9
  10X-33X/RConn1 -- 10X (PLATE)/RConn10
  10X-40X/RConn1 -- 10X (PLATE)/RConn11
  10X-41X/RConn1 -- 10X (PLATE)/RConn12
  10X-42X/RConn1 -- 10X (PLATE)/RConn13
  10X-43X/RConn1 -- 10X (PLATE)/RConn14
  10X-44X/RConn1 -- 10X (PLATE)/RConn15
  10X-45X/RConn1 -- 10X (PLATE)/RConn16
  10X-50X/RConn1 -- 10X (PLATE)/RConn17
  10X-51X/RConn1 -- 10X (PLATE)/RConn18
  10X-52X/RConn1 -- 10X (PLATE)/RConn19
  10X-53X/RConn1 -- 10X (PLATE)/RConn20
  10X-54X/RConn1 -- 10X (PLATE)/RConn21
  10X-55X/RConn1 -- 10X (PLATE)/RConn22
  10X-56X/RConn1 -- 10X (PLATE)/RConn23
  10X-57X/RConn1 -- 10X (PLATE)/RConn24
  10X-58X/RConn1 -- 10X (PLATE)/RConn25
  10X-59X/RConn1 -- 10X (PLATE)/RConn26
  10X-60X/RConn1 -- 10X (PLATE)/RConn27
  10X-61X/RConn1 -- 10X (PLATE)/RConn28
  10X-62X/RConn1 -- 10X (PLATE)/RConn29
  10X-70X/RConn1 -- 10X (PLATE)/RConn30
  10X-71X/RConn1 -- 10X (PLATE)/RConn31
  10X-72X/RConn1 -- 10X (PLATE)/RConn32
  10X-73X/RConn1 -- 10X (PLATE)/RConn33
  10X-74X/RConn1 -- 10X (PLATE)/RConn34

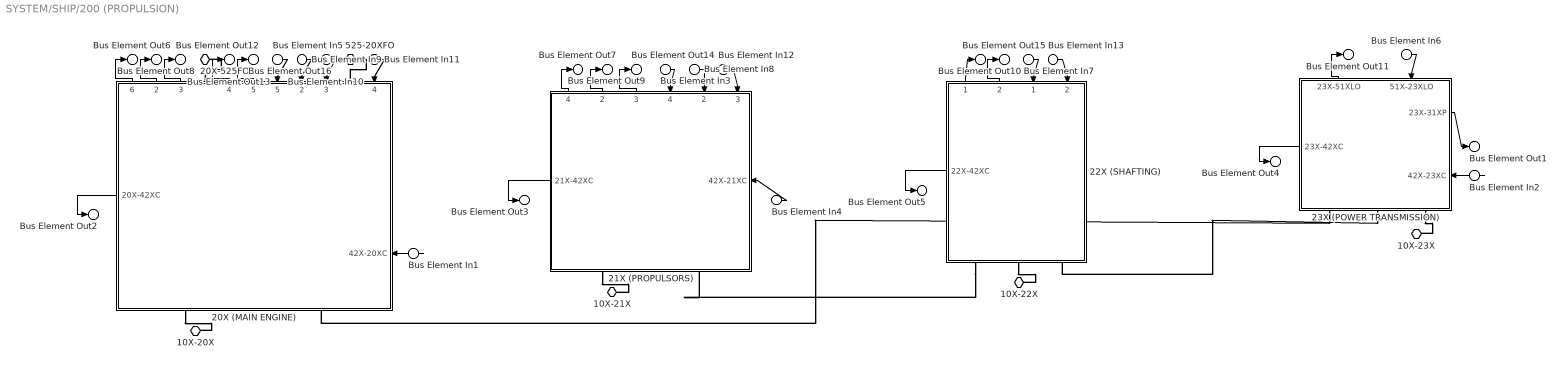
== system SYSTEM/SHIP/200 (PROPULSION) ==
  Bus Element In5 : Inport  PortName=50X-20XCFW
  Bus Element In3 : Inport  Port=2  PortName=50X-21XCFW
  Bus Element In9 : Inport  Port=3  PortName=51X-20XLO
  Bus Element In8 : Inport  Port=4  PortName=51X-21XLO
  Bus Element In7 : Inport  Port=5  PortName=51X-22XLO
  Bus Element In6 : Inport  Port=6  PortName=51X-23XLO
  Bus Element In10 : Inport  Port=7  PortName=52X-20XFO
  Bus Element In11 : Inport  Port=8  PortName=53X-20XCA
  Bus Element In12 : Inport  Port=9  PortName=53X-21XCA
  Bus Element In13 : Inport  Port=10  PortName=53X-22XCA
  Bus Element In1 : Inport  Port=11  PortName=42X-20XC
  Bus Element In4 : Inport  Port=12  PortName=42X-21XC
  Bus Element In2 : Inport  Port=13  PortName=42X-23XC
  20X (MAIN ENGINE) : Subsystem  Variant=on  VariantControlMode=label  LabelModeActiveChoice=20X DIESEL ENGINE
      settings: PortSchema="{\"entries\":[{\"content\":{\"headerSize\":38,\"margin\":15,\"minimumSpacing\":25,\"sides\":[{\"content\":{\"connectorIds\":[\"Out1\"]},\"type\":\"ConnectorPlacement.EquallySpacedRectSide\",\"uuid\":\"c62bca68-e99b-4d4a-8c3b-c9a3c6520291\"},{\"content\":{\"connectorIds\":[\"LConn3\",\"In1\"],\"side\":\"RIGHT\"},\"type\":\"ConnectorPlacement.EquallySpacedRectSide\",\"uuid\":\"9f78cd75-5645-4950-8d66-9f0d33627f1f\"},{\"content\":{\"connectorIds\":[\"Out6\",\"Out2\",\"Out3\",\"LConn1\",\"Out4\",\"Out5\",\"In5\",\"In2\",\"In3\",\"LConn2\",\"In4\"],\"side\":\"TOP\"},\"type\":\"ConnectorPlacement.EquallySpacedRectSide\",\"uuid\":\"f95077c9-4a6b-4bf1-8b13-59697d659817\"},{\"content\":{\"connectorIds\":[\"RConn1\",\"RConn2\"],\"side\":\"BOTTOM\"},\"type\":\"ConnectorPlacement.EquallySpacedRectSide\",\"uuid\":\"0eafd906-a166-4c55-8e00-9a076c1e2d64\"}]},\"type\":\"ConnectorPlacement.EquallySpacedConnector\",\"uuid\":\"da1ef182-4ed3-4fb4-823f-e8eb0a5ecd15\"}],\"packageUris\":[\"http://schema.mathworks.com/mf0/Connector/R2020b\"],\"version\":\"1.0\"}"
  21X (PROPULSORS) : Subsystem  Variant=on  VariantControlMode=label  LabelModeActiveChoice=21X SHAFT DRIVE + MANUVERING THRUSTER
      settings: PortSchema="{\"entries\":[{\"content\":{\"headerSize\":38,\"margin\":15,\"minimumSpacing\":25,\"sides\":[{\"content\":{\"connectorIds\":[\"Out1\"]},\"type\":\"ConnectorPlacement.EquallySpacedRectSide\",\"uuid\":\"c62bca68-e99b-4d4a-8c3b-c9a3c6520291\"},{\"content\":{\"connectorIds\":[\"In1\"],\"side\":\"RIGHT\"},\"type\":\"ConnectorPlacement.EquallySpacedRectSide\",\"uuid\":\"9f78cd75-5645-4950-8d66-9f0d33627f1f\"},{\"content\":{\"connectorIds\":[\"Out4\",\"Out2\",\"Out3\",\"In4\",\"In2\",\"In3\"],\"side\":\"TOP\"},\"type\":\"ConnectorPlacement.EquallySpacedRectSide\",\"uuid\":\"f95077c9-4a6b-4bf1-8b13-59697d659817\"},{\"content\":{\"connectorIds\":[\"RConn1\",\"RConn2\"],\"side\":\"BOTTOM\"},\"type\":\"ConnectorPlacement.EquallySpacedRectSide\",\"uuid\":\"6b5f2b68-9ed2-4485-9686-f8a23585a666\"}]},\"type\":\"ConnectorPlacement.EquallySpacedConnector\",\"uuid\":\"da1ef182-4ed3-4fb4-823f-e8eb0a5ecd15\"}],\"packageUris\":[\"http://schema.mathworks.com/mf0/Connector/R2020b\"],\"version\":\"1.0\"}"
  22X (SHAFTING) : Subsystem  Variant=on  VariantControlMode=label  LabelModeActiveChoice=22X MECHANICAL
      settings: PortSchema="{\"entries\":[{\"content\":{\"headerSize\":38,\"margin\":15,\"minimumSpacing\":25,\"sides\":[{\"content\":{\"connectorIds\":[\"Out3\"]},\"type\":\"ConnectorPlacement.EquallySpacedRectSide\",\"uuid\":\"c62bca68-e99b-4d4a-8c3b-c9a3c6520291\"},{\"content\":{\"side\":\"RIGHT\"},\"type\":\"ConnectorPlacement.EquallySpacedRectSide\",\"uuid\":\"9f78cd75-5645-4950-8d66-9f0d33627f1f\"},{\"content\":{\"connectorIds\":[\"Out1\",\"Out2\",\"In1\",\"In2\"],\"side\":\"TOP\"},\"type\":\"ConnectorPlacement.EquallySpacedRectSide\",\"uuid\":\"f95077c9-4a6b-4bf1-8b13-59697d659817\"},{\"content\":{\"connectorIds\":[\"RConn3\",\"RConn2\",\"RConn1\"],\"side\":\"BOTTOM\"},\"type\":\"ConnectorPlacement.EquallySpacedRectSide\",\"uuid\":\"1f93f758-4269-498d-aa3c-a1654d57bbcc\"}]},\"type\":\"ConnectorPlacement.EquallySpacedConnector\",\"uuid\":\"da1ef182-4ed3-4fb4-823f-e8eb0a5ecd15\"}],\"packageUris\":[\"http://schema.mathworks.com/mf0/Connector/R2020b\"],\"version\":\"1.0\"}"
  23X (POWER TRANSMISSION) : Subsystem  Variant=on  VariantControlMode=label  LabelModeActiveChoice=23X MECHANICAL WITH POWER TAKEOFF
      settings: PortSchema="{\"entries\":[{\"content\":{\"headerSize\":38,\"margin\":15,\"minimumSpacing\":25,\"sides\":[{\"content\":{\"connectorIds\":[\"Out2\"]},\"type\":\"ConnectorPlacement.EquallySpacedRectSide\",\"uuid\":\"c62bca68-e99b-4d4a-8c3b-c9a3c6520291\"},{\"content\":{\"connectorIds\":[\"Out3\",\"In2\"],\"side\":\"RIGHT\"},\"type\":\"ConnectorPlacement.EquallySpacedRectSide\",\"uuid\":\"9f78cd75-5645-4950-8d66-9f0d33627f1f\"},{\"content\":{\"connectorIds\":[\"Out1\",\"In1\"],\"side\":\"TOP\"},\"type\":\"ConnectorPlacement.EquallySpacedRectSide\",\"uuid\":\"f95077c9-4a6b-4bf1-8b13-59697d659817\"},{\"content\":{\"connectorIds\":[\"LConn2\",\"LConn1\",\"RConn1\"],\"side\":\"BOTTOM\"},\"type\":\"ConnectorPlacement.EquallySpacedRectSide\",\"uuid\":\"886e986c-d088-4ccd-a11a-30cba32770e8\"}]},\"type\":\"ConnectorPlacement.EquallySpacedConnector\",\"uuid\":\"da1ef182-4ed3-4fb4-823f-e8eb0a5ecd15\"}],\"packageUris\":[\"http://schema.mathworks.com/mf0/Connector/R2020b\"],\"version\":\"1.0\"}"
  20X-525FO : PMIOPort  Side=Left  ConnectionType=Bus: FuelOil_P
  525-20XFO : PMIOPort  Port=2  Side=Left  ConnectionType=Bus: FuelOil_P
  10X-20X : PMIOPort  Port=3  Side=Left  ConnectionType=Bus: Physical
  10X-21X : PMIOPort  Port=4  Side=Left  ConnectionType=Bus: Physical
  10X-22X : PMIOPort  Port=5  Side=Left  ConnectionType=Bus: Physical
  10X-23X : PMIOPort  Port=6  Side=Left  ConnectionType=Bus: Physical
  Bus Element Out6 : Outport  PortName=20X-50XCFW
  Bus Element Out8 : Outport  Port=2  PortName=20X-51XLO
  Bus Element Out12 : Outport  Port=3  PortName=20X-52XFO
  Bus Element Out13 : Outport  Port=4  PortName=20X-53XCA
  Bus Element Out16 : Outport  Port=5  PortName=20X-57XWG
  Bus Element Out7 : Outport  Port=6  PortName=21X-50XCFW
  Bus Element Out9 : Outport  Port=7  PortName=21X-51XLO
  Bus Element Out14 : Outport  Port=8  PortName=21X-53XCA
  Bus Element Out10 : Outport  Port=9  PortName=22X-51XLO
  Bus Element Out15 : Outport  Port=10  PortName=22X-53XCA
  Bus Element Out11 : Outport  Port=11  PortName=23X-51XLO
  Bus Element Out2 : Outport  Port=12  PortName=20X-42XC
  Bus Element Out3 : Outport  Port=13  PortName=21X-42XC
  Bus Element Out5 : Outport  Port=14  PortName=22X-42XC
  Bus Element Out4 : Outport  Port=15  PortName=23X-42XC
  Bus Element Out1 : Outport  Port=16  PortName=23X-31XP
  wires:
  Bus Element In1/1 -> 20X (MAIN ENGINE)/1(42X-20XC)
  Bus Element In9/1 -> 20X (MAIN ENGINE)/2(51X-20XLO)
  Bus Element In10/1 -> 20X (MAIN ENGINE)/3(52X-20XFO)
  Bus Element In11/1 -> 20X (MAIN ENGINE)/4(53X-20XCA)
  Bus Element In5/1 -> 20X (MAIN ENGINE)/5(50X-20XCFW)
  20X (MAIN ENGINE)/1(20X-42XC) -> Bus Element Out2/1
  20X (MAIN ENGINE)/2(20X-51XLO) -> Bus Element Out8/1
  20X (MAIN ENGINE)/3(20X-52XFO) -> Bus Element Out12/1
  20X (MAIN ENGINE)/4(20X-53XCA) -> Bus Element Out13/1
  20X (MAIN ENGINE)/5(20X-57XWG) -> Bus Element Out16/1
  20X (MAIN ENGINE)/6(20X-50XCFW) -> Bus Element Out6/1
  Bus Element In4/1 -> 21X (PROPULSORS)/1(42X-21XC)
  Bus Element In8/1 -> 21X (PROPULSORS)/2(51X-21XLO)
  Bus Element In12/1 -> 21X (PROPULSORS)/3(53X-21XCA)
  Bus Element In3/1 -> 21X (PROPULSORS)/4(50X-21XCFW)
  21X (PROPULSORS)/1(21X-42XC) -> Bus Element Out3/1
  21X (PROPULSORS)/2(21X-51XLO) -> Bus Element Out9/1
  21X (PROPULSORS)/3(21X-53XCA) -> Bus Element Out14/1
  21X (PROPULSORS)/4(21X-50XCFW) -> Bus Element Out7/1
  Bus Element In7/1 -> 22X (SHAFTING)/1(51X-22XLO)
  Bus Element In13/1 -> 22X (SHAFTING)/2(53X-22XCA)
  22X (SHAFTING)/1(22X-51XLO) -> Bus Element Out10/1
  22X (SHAFTING)/2(22X-53XCA) -> Bus Element Out15/1
  22X (SHAFTING)/3(22X-42XC) -> Bus Element Out5/1
  Bus Element In6/1 -> 23X (POWER TRANSMISSION)/1(51X-23XLO)
  Bus Element In2/1 -> 23X (POWER TRANSMISSION)/2(42X-23XC)
  23X (POWER TRANSMISSION)/1(23X-51XLO) -> Bus Element Out11/1
  23X (POWER TRANSMISSION)/2(23X-42XC) -> Bus Element Out4/1
  23X (POWER TRANSMISSION)/3(23X-31XP) -> Bus Element Out1/1
  connections:
  20X (MAIN ENGINE)/LConn1 -- 20X-525FO/RConn1
  20X (MAIN ENGINE)/LConn2 -- 525-20XFO/RConn1
  20X (MAIN ENGINE)/RConn1 -- 10X-20X/RConn1
  21X (PROPULSORS)/RConn1 -- 10X-21X/RConn1
  22X (SHAFTING)/RConn2 -- 10X-22X/RConn1
  22X (SHAFTING)/RConn3 -- 21X (PROPULSORS)/RConn2
  23X (POWER TRANSMISSION)/LConn1 -- 22X (SHAFTING)/RConn1
  23X (POWER TRANSMISSION)/LConn2 -- 20X (MAIN ENGINE)/RConn2
  23X (POWER TRANSMISSION)/RConn1 -- 10X-23X/RConn1
